simulink model "Practica_1_SMS_sim"  (R2022a)
settings: Solver=VariableStepAuto  StartTime=0.0  StopTime=10.0  MaxStep=0.0001  RelTol=1e-3
undefined symbols (not defined in the file): g, l_1, l_2, m1, m2
settings Model: Creator=Peri_XP  LastModifiedBy=Peri_XP

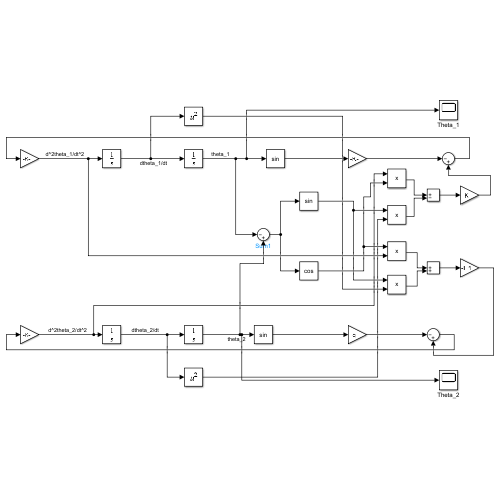
[thumbnail: Simulink's stored preview of the top-level diagram]
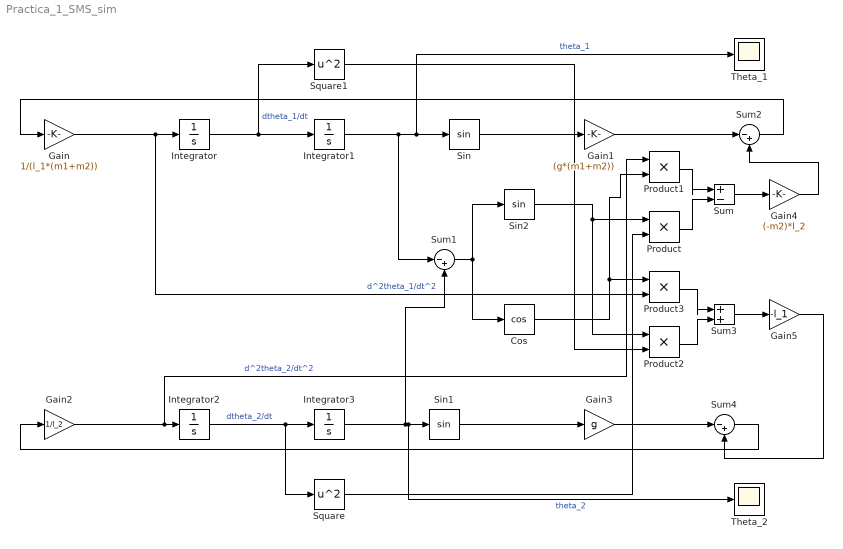
== system Practica_1_SMS_sim ==
  Cos : Trigonometry  Operator=cos
  Gain : Gain  Gain=1/(l_1*(m1+m2))
  Gain1 : Gain  Gain=(g*(m1+m2))
  Gain2 : Gain  Gain=1/l_2
  Gain3 : Gain  Gain=g
  Gain4 : Gain  Gain=(-m2)*l_2
  Gain5 : Gain  Gain=-l_1
  Integrator : Integrator
  Integrator1 : Integrator
  Integrator2 : Integrator
  Integrator3 : Integrator  InitialCondition=(35*pi)/180
  Product{,1..3} (4 alike) : Product
  Sin : Trigonometry
  Sin1 : Trigonometry
  Sin2 : Trigonometry
  Square : Math  Operator=square
  Square1 : Math  Operator=square
  Sum : Sum  Inputs=|+-
  Sum1 : Sum  Inputs=|-+
  Sum2 : Sum  Inputs=|-+
  Sum3 : Sum  Inputs=|++
  Sum4 : Sum  Inputs=|-+
  Theta_1 : Scope
  Theta_2 : Scope
  wires:
  Gain/1 -> Product3/2, Integrator/1  "d^2theta_1/dt^2"
  Integrator/1 -> Square1/1, Integrator1/1  "dtheta_1/dt"
  Integrator1/1 -> Sum1/1, Theta_1/1, Sin/1  "theta_1"
  Sin/1 -> Gain1/1
  Gain2/1 -> Product1/1, Integrator2/1  "d^2theta_2/dt^2"
  Integrator2/1 -> Square/1, Integrator3/1  "dtheta_2/dt"
  Integrator3/1 -> Sum1/2, Theta_2/1, Sin1/1  "theta_2"
  Sin1/1 -> Gain3/1
  Sum1/1 -> Cos/1, Sin2/1
  Sin2/1 -> Product2/1, Product/1
  Cos/1 -> Product1/2, Product3/1
  Product1/1 -> Sum/1
  Product/1 -> Sum/2
  Square/1 -> Product/2
  Gain1/1 -> Sum2/1
  Sum/1 -> Gain4/1
  Gain4/1 -> Sum2/2
  Sum2/1 -> Gain/1
  Square1/1 -> Product2/2
  Product3/1 -> Sum3/1
  Product2/1 -> Sum3/2
  Sum3/1 -> Gain5/1
  Gain3/1 -> Sum4/1
  Gain5/1 -> Sum4/2
  Sum4/1 -> Gain2/1
